simulink model "Mission_Server_Swarm_2QDrone_FrSky"  (Simulink 10.1)
settings: Solver=ode2  StartTime=0.0  StopTime=inf  FixedStep=0.001  RelTol=1e-3  EnableMultiTasking=on
undefined symbols (not defined in the file): datetime, Host, m, qc_get_step_size, saved_data
libraries: quarc_library x33, simulink x7
(part 2 of 2)

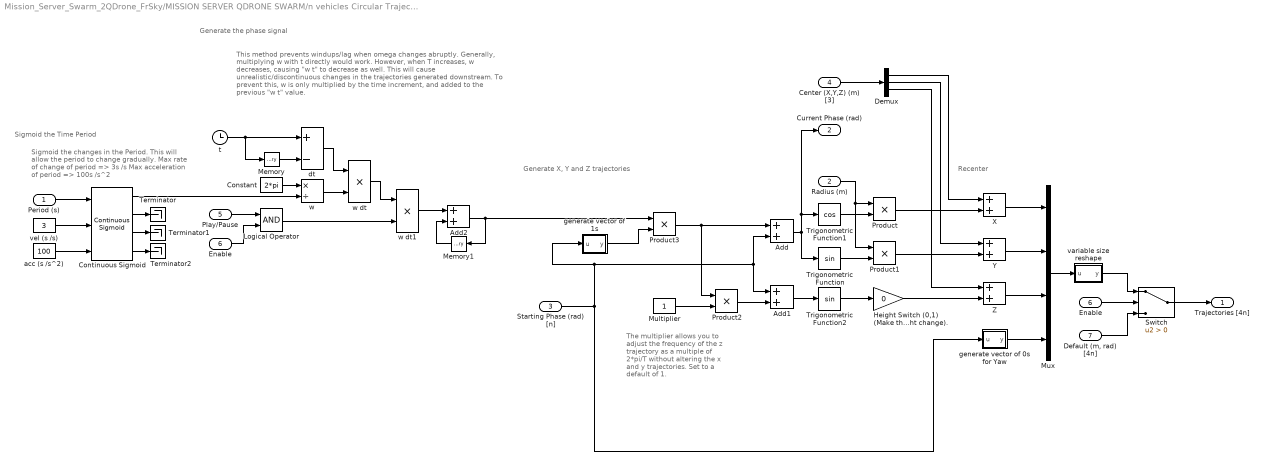
== system Mission_Server_Swarm_2QDrone_FrSky/MISSION SERVER QDRONE SWARM/n vehicles Circular Trajectories ==
  note: Recenter
  note: Generate X, Y and Z trajectories
  note: Generate the phase signal
  note: Sigmoid the changes in the Period. This will
      | allow the period to change gradually.
      | Max rate of change of period => 3s /s
      | Max acceleration of period => 100s /s^2
  note: Sigmoid the Time Period
  note: The multiplier allows you to adjust the frequency of the z trajectory as a multiple of 2*pi/T without altering the x and y trajectories. Set to a default of 1.
  note: This method prevents windups/lag when omega changes abruptly. Generally, multiplying w with t directly would work. However, when T increases, w decreases, causing "w t" to decrease as well. This will cause unrealistic/discontinuous changes in the trajectories generated downstream.
      |
      | To prevent this, w is only multiplied by the time increment, and added to the previous "w t" value.
  Period (s) : Inport
  Radius (m) : Inport  Port=2
  Starting Phase (rad) [n] : Inport  Port=3
  Center (X,Y,Z) (m) [3] : Inport  Port=4
  Play/Pause : Inport  Port=5
  Enable : Inport  Port=6
  "Default (m, rad) [4n]" : Inport  Port=7
  " Enable " : InportShadow  Port=6
  Add : Sum
  Add1 : Sum
  Add2 : Sum
  Constant : Constant  Value=2*pi
  Continuous Sigmoid : quarc_library/Sources/Sigmoids/Continuous Sigmoid  params_source=External (input ports)  max_velocity=2  max_acceleration=10  initial_position=10  initial_velocity=0  hold_off=0.5  input_sample_time=-1  output_sample_time=qc_get_step_size
      settings: SourceProductName=QUARC Targets
  Demux : Demux  Outputs=3
  Height Switch (0,1) (Make this 0 to disable height change). : Gain  Gain=0
  Logical Operator : Logic  AllPortsSameDT=off  OutDataTypeStr=boolean
  Memory : Memory
  Memory1 : Memory
  Multiplier : Constant
  Mux : Mux
  Product{,1..3} (4 alike) : Product
  Switch : Switch  Criteria=u2 > Threshold
  Terminator : Terminator
  Terminator1 : Terminator
  Terminator2 : Terminator
  Trigonometric Function : Trigonometry
  Trigonometric Function1 : Trigonometry  Operator=cos
  Trigonometric Function2 : Trigonometry
  X : Sum
  Y : Sum
  Z : Sum
  acc (s /s^2) : Constant  Value=100
  dt : Sum  Inputs=+-
  generate vector of 0s for Yaw : MATLAB Function  TreatAsAtomicUnit=on
  generate vector of 1s : MATLAB Function  TreatAsAtomicUnit=on
  t : Clock
  variable size reshape : MATLAB Function  TreatAsAtomicUnit=on
  vel (s /s) : Constant  Value=3
  w : Product  Inputs=*/
  w dt : Product
  w dt1 : Product
  Trajectories [4n] : Outport  VectorParamsAs1DForOutWhenUnconnected=off
  Current Phase (rad) : Outport  Port=2  VectorParamsAs1DForOutWhenUnconnected=off
  wires:
  Trigonometric Function/1 -> Product1/2
  Trigonometric Function1/1 -> Product/2
  Height Switch (0,1) (Make this 0 to disable height change)./1 -> Z/2
  Product1/1 -> Y/2
  Product/1 -> X/2
  Radius (m)/1 -> Product/1, Product1/1
  generate vector of 0s for Yaw/1(y) -> Mux/4
  Continuous Sigmoid/4 -> Terminator2/1
  Period (s)/1 -> Continuous Sigmoid/1
  Continuous Sigmoid/2 -> Terminator/1
  Continuous Sigmoid/3 -> Terminator1/1
  acc (s /s^2)/1 -> Continuous Sigmoid/3
  vel (s /s)/1 -> Continuous Sigmoid/2
  Add1/1 -> Trigonometric Function2/1
  Multiplier/1 -> Product2/2
  Starting Phase (rad) [n]/1 -> generate vector of 1s/1(u), Add/2, Add1/1, generate vector of 0s for Yaw/1(u)
  Add2/1 -> Product3/1, Memory1/1
  Add/1 -> Current Phase (rad)/1, Trigonometric Function1/1, Trigonometric Function/1
  Center (X,Y,Z) (m) [3]/1 -> Demux/1
  Demux/2 -> Y/1
  Demux/1 -> X/1
  Trigonometric Function2/1 -> Height Switch (0,1) (Make this 0 to disable height change)./1
  Demux/3 -> Z/1
  X/1 -> Mux/1
  Y/1 -> Mux/2
  Z/1 -> Mux/3
  Memory/1 -> dt/2
  w dt/1 -> w dt1/1
  w dt1/1 -> Add2/1
  Constant/1 -> w/1
  Memory1/1 -> Add2/2
  w/1 -> w dt/2
  Continuous Sigmoid/1 -> w/2
  t/1 -> Memory/1, dt/1
  dt/1 -> w dt/1
  Mux/1 -> variable size reshape/1(u)
  Switch/1 -> Trajectories [4n]/1
  "Default (m, rad) [4n]"/1 -> Switch/3
  Enable/1 -> Switch/2
  Play/Pause/1 -> Logical Operator/1
  " Enable "/1 -> Logical Operator/2
  Logical Operator/1 -> w dt1/2
  Product3/1 -> Add/1, Product2/1
  variable size reshape/1(y) -> Switch/1
  generate vector of 1s/1(y) -> Product3/2
  Product2/1 -> Add1/2

== system Mission_Server_Swarm_2QDrone_FrSky/MISSION SERVER QDRONE SWARM/Calculate Home Pose V1/Enabled Subsystem ==
  "Pose (m, rad ) [4] " : Inport
  Enable : EnablePort
  "Home Pose (m, rad ) [4]" : Outport  VectorParamsAs1DForOutWhenUnconnected=off
  wires:
  "Pose (m, rad ) [4] "/1 -> "Home Pose (m, rad ) [4]"/1

== system Mission_Server_Swarm_2QDrone_FrSky/MISSION SERVER QDRONE SWARM/Calculate Home Pose V2/Enabled Subsystem ==
  "Pose (m, rad ) [4] " : Inport
  Enable : EnablePort
  "Home Pose (m, rad ) [4]" : Outport  VectorParamsAs1DForOutWhenUnconnected=off
  wires:
  "Pose (m, rad ) [4] "/1 -> "Home Pose (m, rad ) [4]"/1

== system Mission_Server_Swarm_2QDrone_FrSky/MISSION SERVER QDRONE SWARM/Calculate Home Pose V7/Enabled Subsystem ==
  "Pose (m, rad ) [4] " : Inport
  Enable : EnablePort
  "Home Pose (m, rad ) [4]" : Outport  VectorParamsAs1DForOutWhenUnconnected=off
  wires:
  "Pose (m, rad ) [4] "/1 -> "Home Pose (m, rad ) [4]"/1

== system Mission_Server_Swarm_2QDrone_FrSky/MISSION SERVER QDRONE SWARM/Communications Check/Triggered Subsystem ==
  note: This looks for the first falling edge to trigger a communication issue,
      | because the mission server model starts first.
  Trigger : TriggerPort  TriggerType=falling  VariantControl=Variant
  Add : Sum
  Compare To Constant : simulink/Logic and Bit Operations/Compare To Constant  relop=>=  const=1  OutDataTypeStr=boolean
  Constant : Constant
  Memory : Memory  InheritSampleTime=on
  Communication Issue (0,1) : Outport  InitialOutput=0  VectorParamsAs1DForOutWhenUnconnected=off
  wires:
  Constant/1 -> Add/1
  Memory/1 -> Add/2
  Add/1 -> Compare To Constant/1, Memory/1
  Compare To Constant/1 -> Communication Issue (0,1)/1

== system Mission_Server_Swarm_2QDrone_FrSky/MISSION SERVER QDRONE SWARM/Communications Check/Triggered Subsystem1 ==
  note: This looks for the first falling edge to trigger a communication issue,
      | because the mission server model starts first.
  Trigger : TriggerPort  TriggerType=falling  VariantControl=Variant
  Add : Sum
  Compare To Constant : simulink/Logic and Bit Operations/Compare To Constant  relop=>=  const=1  OutDataTypeStr=boolean
  Constant : Constant
  Memory : Memory  InheritSampleTime=on
  Communication Issue (0,1) : Outport  InitialOutput=0  VectorParamsAs1DForOutWhenUnconnected=off
  wires:
  Compare To Constant/1 -> Communication Issue (0,1)/1
  Add/1 -> Memory/1, Compare To Constant/1
  Memory/1 -> Add/2
  Constant/1 -> Add/1

== system Mission_Server_Swarm_2QDrone_FrSky/MISSION SERVER QDRONE SWARM/Data Server (Localization) /Convention Correction (Motive Frame to Research Studio Frame) - Drone 1 ==
  note: MF_R_RSF
  note: This subsystem converts measurements in the Motive Frame (MF)(raw optitrack) into the Research Studio Frame (RSF).
  note: RSF_R_MF
  note: XYZ in MF
  note: RPY in MF
  note: position
  note: attitude
  note: XYZ in RSF
  note: RPY in RSF
  xyz_MF (m) [3] : Inport
  rot_MF (rad) [3] : Inport  Port=2
  Inverse of  Orthonormal  Matrix is its  Transpose : Math  Operator=transpose  SignedPower=on  SaturateOnIntegerOverflow=on
  Prevent Gimbal Lock : Subsystem
  Product : Product  Multiplication=Matrix(*)
  Product1 : Product  Multiplication=Matrix(*)
  Rotate Basis from  RSF to MF : Constant  Value=[0 -1 0;0 0 1;-1 0 0]
  xyz_RSF (m) [3] : Outport  VectorParamsAs1DForOutWhenUnconnected=off
  rot_RSF (rad) [3] : Outport  Port=2  VectorParamsAs1DForOutWhenUnconnected=off
  wires:
  Rotate Basis from  RSF to MF/1 -> Inverse of  Orthonormal  Matrix is its  Transpose/1
  xyz_MF (m) [3]/1 -> Product1/2
  Inverse of  Orthonormal  Matrix is its  Transpose/1 -> Product1/1, Product/1
  rot_MF (rad) [3]/1 -> Product/2
  Product1/1 -> xyz_RSF (m) [3]/1
  Product/1 -> Prevent Gimbal Lock/1(Attitude (rad) [3])
  Prevent Gimbal Lock/1("Attitude (rad) [3] ") -> rot_RSF (rad) [3]/1

== system Mission_Server_Swarm_2QDrone_FrSky/MISSION SERVER QDRONE SWARM/Data Server (Localization) /Convention Correction (Motive Frame to Research Studio Frame) - Drone 2 ==
  note: RPY in RSF
  note: XYZ in RSF
  note: attitude
  note: position
  note: RPY in MF
  note: XYZ in MF
  note: RSF_R_MF
  note: This subsystem converts measurements in the Motive Frame (MF)(raw optitrack) into the Research Studio Frame (RSF).
  note: MF_R_RSF
  xyz_MF (m) [3] : Inport
  rot_MF (rad) [3] : Inport  Port=2
  Inverse of  Orthonormal  Matrix is its  Transpose : Math  Operator=transpose  SignedPower=on  SaturateOnIntegerOverflow=on
  Prevent Gimbal Lock : Subsystem
  Product : Product  Multiplication=Matrix(*)
  Product1 : Product  Multiplication=Matrix(*)
  Rotate Basis from  RSF to MF : Constant  Value=[0 -1 0;0 0 1;-1 0 0]
  xyz_RSF (m) [3] : Outport  VectorParamsAs1DForOutWhenUnconnected=off
  rot_RSF (rad) [3] : Outport  Port=2  VectorParamsAs1DForOutWhenUnconnected=off
  wires:
  Prevent Gimbal Lock/1("Attitude (rad) [3] ") -> rot_RSF (rad) [3]/1
  Product/1 -> Prevent Gimbal Lock/1(Attitude (rad) [3])
  Product1/1 -> xyz_RSF (m) [3]/1
  rot_MF (rad) [3]/1 -> Product/2
  Inverse of  Orthonormal  Matrix is its  Transpose/1 -> Product/1, Product1/1
  xyz_MF (m) [3]/1 -> Product1/2
  Rotate Basis from  RSF to MF/1 -> Inverse of  Orthonormal  Matrix is its  Transpose/1

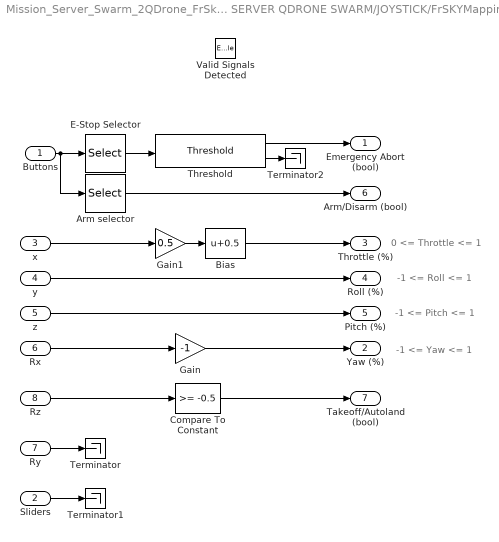
== system Mission_Server_Swarm_2QDrone_FrSky/MISSION SERVER QDRONE SWARM/JOYSTICK/FrSKYMapping ==
  note: -1 <= Pitch <= 1
  note: -1 <= Roll <= 1
  note: 0 <= Throttle <= 1
  note: -1 <= Yaw <= 1
  Buttons : Inport
  Sliders : Inport  Port=2
  x : Inport  Port=3
  y : Inport  Port=4
  z : Inport  Port=5
  Rx : Inport  Port=6
  Ry : Inport  Port=7
  Rz : Inport  Port=8
  Valid Signals Detected : EnablePort
  Arm selector : Selector  InputPortWidth=32  IndexOptions=Index vector (dialog)  Indices=[2]  OutputSizes=1
  Bias : Bias  Bias=0.5
  Compare To Constant : simulink/Logic and Bit Operations/Compare To Constant  relop=>=  const=-0.5  OutDataTypeStr=boolean
  E-Stop Selector : Selector  InputPortWidth=32  IndexOptions=Index vector (dialog)  Indices=[1]  OutputSizes=1
  Gain : Gain  Gain=-1
  Gain1 : Gain  Gain=0.5
  Terminator : Terminator
  Terminator1 : Terminator
  Terminator2 : Terminator
  Threshold : quarc_library/Discontinuities/Threshold  operator=>=  param_src=Specify via dialog  threshold=0.5  duration=0.2
      settings: SourceProductName=QUARC Targets
  Emergency Abort (bool) : Outport  VectorParamsAs1DForOutWhenUnconnected=off
  Yaw (%) : Outport  Port=2  VectorParamsAs1DForOutWhenUnconnected=off
  Throttle (%) : Outport  Port=3  VectorParamsAs1DForOutWhenUnconnected=off
  Roll (%) : Outport  Port=4  VectorParamsAs1DForOutWhenUnconnected=off
  Pitch (%) : Outport  Port=5  VectorParamsAs1DForOutWhenUnconnected=off
  "Arm/Disarm (bool) " : Outport  Port=6  VectorParamsAs1DForOutWhenUnconnected=off
  Takeoff/Autoland (bool) : Outport  Port=7  VectorParamsAs1DForOutWhenUnconnected=off
  wires:
  Bias/1 -> Throttle (%)/1
  Gain1/1 -> Bias/1
  Gain/1 -> Yaw (%)/1
  Threshold/2 -> Terminator2/1
  Threshold/1 -> Emergency Abort (bool)/1
  Compare To Constant/1 -> Takeoff/Autoland (bool)/1
  Rz/1 -> Compare To Constant/1
  E-Stop Selector/1 -> Threshold/1
  Sliders/1 -> Terminator1/1
  Ry/1 -> Terminator/1
  Rx/1 -> Gain/1
  z/1 -> Pitch (%)/1
  y/1 -> Roll (%)/1
  x/1 -> Gain1/1
  Arm selector/1 -> "Arm/Disarm (bool) "/1
  Buttons/1 -> E-Stop Selector/1, Arm selector/1

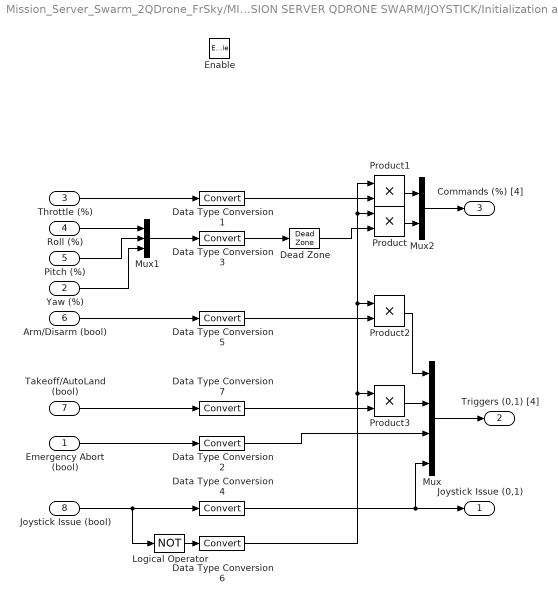
== system Mission_Server_Swarm_2QDrone_FrSky/MISSION SERVER QDRONE SWARM/JOYSTICK/Initialization and Conditioning ==
  Emergency Abort (bool) : Inport
  Yaw (%) : Inport  Port=2
  Throttle (%) : Inport  Port=3
  Roll (%) : Inport  Port=4
  Pitch (%) : Inport  Port=5
  Arm/Disarm (bool) : Inport  Port=6
  Takeoff/AutoLand (bool) : Inport  Port=7
  Joystick Issue (bool) : Inport  Port=8
  Enable : EnablePort  StatesWhenEnabling=reset
  Data Type Conversion{1..7} (7 alike) : DataTypeConversion
  Dead Zone : DeadZone  LowerValue=-0.01  UpperValue=0.01  SaturateOnIntegerOverflow=on
  Logical Operator : Logic  Operator=NOT  AllPortsSameDT=off  OutDataTypeStr=boolean
  Mux : Mux
  Mux1 : Mux  Inputs=3
  Mux2 : Mux  Inputs=2
  Product{,1..3} (4 alike) : Product
  Joystick Issue (0,1) : Outport  InitialOutput=0  VectorParamsAs1DForOutWhenUnconnected=off
  Triggers (0,1) [4] : Outport  Port=2  InitialOutput=0  VectorParamsAs1DForOutWhenUnconnected=off
  Commands (%) [4] : Outport  Port=3  InitialOutput=0  VectorParamsAs1DForOutWhenUnconnected=off
  wires:
  Mux2/1 -> Commands (%) [4]/1
  Data Type Conversion7/1 -> Product3/2
  Product3/1 -> Mux/2
  Takeoff/AutoLand (bool)/1 -> Data Type Conversion7/1
  Data Type Conversion5/1 -> Product2/2
  Product2/1 -> Mux/1
  Data Type Conversion6/1 -> Product3/1, Product2/1, Product/1, Product1/1
  Dead Zone/1 -> Product/2
  Data Type Conversion1/1 -> Product1/2
  Product1/1 -> Mux2/1
  Product/1 -> Mux2/2
  Logical Operator/1 -> Data Type Conversion6/1
  Data Type Conversion2/1 -> Mux/3
  Mux/1 -> Triggers (0,1) [4]/1
  Arm/Disarm (bool)/1 -> Data Type Conversion5/1
  Data Type Conversion3/1 -> Dead Zone/1
  Emergency Abort (bool)/1 -> Data Type Conversion2/1
  Data Type Conversion4/1 -> Joystick Issue (0,1)/1, Mux/4
  Yaw (%)/1 -> Mux1/3
  Pitch (%)/1 -> Mux1/2
  Roll (%)/1 -> Mux1/1
  Throttle (%)/1 -> Data Type Conversion1/1
  Mux1/1 -> Data Type Conversion3/1
  Joystick Issue (bool)/1 -> Logical Operator/1, Data Type Conversion4/1

== system Mission_Server_Swarm_2QDrone_FrSky/MISSION SERVER QDRONE SWARM/JOYSTICK/Pulse Check ==
  note: For this subsystem we will count the number of new pulses. The data can be considered enabled once the count of new signals has gone beyond 1. This will enable the Initializing and conditioning subsystem.
  new : Inport
  Compare : quarc_library/Logic Operations/Compare  operator=>=  output_data_type=boolean
      settings: SourceProductName=QUARC Targets
  Pulse Check : Constant
  "pulse count " : Subsystem  TreatAsAtomicUnit=on
  signal enable : Outport  InitialOutput=0  VectorParamsAs1DForOutWhenUnconnected=off
  wires:
  Compare/1 -> signal enable/1
  Pulse Check/1 -> Compare/2
  new/1 -> "pulse count "/Trigger
  "pulse count "/1(Number of Pulses) -> Compare/1

== system Mission_Server_Swarm_2QDrone_FrSky/MISSION SERVER QDRONE SWARM/Data Server (Localization) /Convention Correction (Motive Frame to Research Studio Frame) - Drone 1/Prevent Gimbal Lock ==
  note: Remapping the rotation order to prevent gimbal lock
      | in heading/yaw due to Euler singularity condition
  Attitude (rad) [3] : Inport
  Demux : Demux  Outputs=3
  Euler Angles from Rotation Matrix (Relative ZYX) : quarc_library/Math Operations/Matrices/Euler Angles from Rotation Matrix  menu_order=Relative Z-Y-X
      settings: SourceProductName=QUARC Targets
  Euler Angles to Rotation Matrix (Relative YZX) : quarc_library/Math Operations/Matrices/Euler Angles to Rotation Matrix  menu_order=Relative Y-Z-X
      settings: SourceProductName=QUARC Targets
  Mux : Mux  Inputs=3
  "Attitude (rad) [3] " : Outport  VectorParamsAs1DForOutWhenUnconnected=off
  wires:
  Euler Angles from Rotation Matrix (Relative ZYX)/2 -> Mux/2
  Euler Angles from Rotation Matrix (Relative ZYX)/1 -> Mux/3
  Euler Angles from Rotation Matrix (Relative ZYX)/3 -> Mux/1
  Euler Angles to Rotation Matrix (Relative YZX)/1 -> Euler Angles from Rotation Matrix (Relative ZYX)/1
  Attitude (rad) [3]/1 -> Demux/1
  Mux/1 -> "Attitude (rad) [3] "/1
  Demux/2 -> Euler Angles to Rotation Matrix (Relative YZX)/1
  Demux/3 -> Euler Angles to Rotation Matrix (Relative YZX)/2
  Demux/1 -> Euler Angles to Rotation Matrix (Relative YZX)/3

== system Mission_Server_Swarm_2QDrone_FrSky/MISSION SERVER QDRONE SWARM/Data Server (Localization) /Convention Correction (Motive Frame to Research Studio Frame) - Drone 2/Prevent Gimbal Lock ==
  note: Remapping the rotation order to prevent gimbal lock
      | in heading/yaw due to Euler singularity condition
  Attitude (rad) [3] : Inport
  Demux : Demux  Outputs=3
  Euler Angles from Rotation Matrix (Relative ZYX) : quarc_library/Math Operations/Matrices/Euler Angles from Rotation Matrix  menu_order=Relative Z-Y-X
      settings: SourceProductName=QUARC Targets
  Euler Angles to Rotation Matrix (Relative YZX) : quarc_library/Math Operations/Matrices/Euler Angles to Rotation Matrix  menu_order=Relative Y-Z-X
      settings: SourceProductName=QUARC Targets
  Mux : Mux  Inputs=3
  "Attitude (rad) [3] " : Outport  VectorParamsAs1DForOutWhenUnconnected=off
  wires:
  Demux/1 -> Euler Angles to Rotation Matrix (Relative YZX)/3
  Demux/3 -> Euler Angles to Rotation Matrix (Relative YZX)/2
  Demux/2 -> Euler Angles to Rotation Matrix (Relative YZX)/1
  Mux/1 -> "Attitude (rad) [3] "/1
  Attitude (rad) [3]/1 -> Demux/1
  Euler Angles to Rotation Matrix (Relative YZX)/1 -> Euler Angles from Rotation Matrix (Relative ZYX)/1
  Euler Angles from Rotation Matrix (Relative ZYX)/3 -> Mux/1
  Euler Angles from Rotation Matrix (Relative ZYX)/1 -> Mux/3
  Euler Angles from Rotation Matrix (Relative ZYX)/2 -> Mux/2

== system Mission_Server_Swarm_2QDrone_FrSky/MISSION SERVER QDRONE SWARM/JOYSTICK/Pulse Check/pulse count  ==
  Trigger : TriggerPort  TriggerType=either  VariantControl=Variant
  Constant1 : Constant  Value=0
  Increment Stored Integer : simulink/Additional Math & Discrete/Additional Math: Increment - Decrement/Increment Stored Integer
  Sum : Sum  Inputs=|++
  Unit Delay : UnitDelay  SampleTime=-1  HasFrameUpgradeWarning=on
  Number of Pulses : Outport  VectorParamsAs1DForOutWhenUnconnected=off
  wires:
  Constant1/1 -> Sum/1
  Sum/1 -> Increment Stored Integer/1
  Unit Delay/1 -> Sum/2
  Increment Stored Integer/1 -> Unit Delay/1, Number of Pulses/1

== matlab function MISSION SERVER QDRONE SWARM/n vehicles Circular Trajectories/generate vector of 0s for Yaw ==
  data: u input double; y output double
function y = fcn(u)

y = 0.*u;

== matlab function MISSION SERVER QDRONE SWARM/n vehicles Circular Trajectories/generate vector of 1s ==
  data: u input double; y output double
function y = fcn(u)

y = 0.*u + 1;

== matlab function MISSION SERVER QDRONE SWARM/n vehicles Circular Trajectories/variable size reshape ==
  data: u input double; y output double
function y = fcn(u)
y = u;
num = length(u)/4;
for i = 1:4
    for j = 1:num
        y(4*(j-1) + i) = u(j + num*(i-1));
    end
end

== matlab function Communication V1/Detect Communication loss/MATLAB Function ==
  data: time input double; stream_connection_loss output double; state input double; error input double
function stream_connection_loss  = fcn(time, state, error)

stream_connection_loss = 0;
if time > 1
    if ~((state == 2)&&(error >= 0))
        % stream connection is not established correctly
        stream_connection_loss = 1;
    end
end

== matlab function Communication V2/Detect Communication loss/MATLAB Function ==
  data: time input double; stream_connection_loss output double; state input double; error input double
function stream_connection_loss  = fcn(time, state, error)

stream_connection_loss = 0;
if time > 1
    if ~((state == 2)&&(error >= 0))
        % stream connection is not established correctly
        stream_connection_loss = 1;
    end
end

== matlab function MISSION SERVER QDRONE SWARM/Extract Vehicle Data 7/Extract Object Data ==
  data: data input double; position output double; orientation output double; index input double; tracking output double
function [position, orientation, tracking] = fcn(data, index)

n = length(data)/7;

if (index<=0)||(index>n)
    position = zeros(1,3); orientation = zeros(1,3); tracking = 0;
else
    position = [data(index*3-2), data(index*3-1), data(index*3)];
    orientation = [data((index+n)*3 - 2), data((index+n)*3 - 1), data((index+n)*3)];
    tracking = data(index + (n*6));
end

== matlab function MISSION SERVER QDRONE SWARM/Extract Vehicle Data 1/Extract Object Data ==
  data: data input double; position output double; orientation output double; index input double; tracking output double
function [position, orientation, tracking] = fcn(data, index)

n = length(data)/7;

if (index<=0)||(index>n)
    position = zeros(1,3); orientation = zeros(1,3); tracking = 0;
else
    position = [data(index*3-2), data(index*3-1), data(index*3)];
    orientation = [data((index+n)*3 - 2), data((index+n)*3 - 1), data((index+n)*3)];
    tracking = data(index + (n*6));
end

== matlab function MISSION SERVER QDRONE SWARM/Extract Vehicle Data 2/Extract Object Data ==
  data: data input double; position output double; orientation output double; index input double; tracking output double
function [position, orientation, tracking] = fcn(data, index)

n = length(data)/7;

if (index<=0)||(index>n)
    position = zeros(1,3); orientation = zeros(1,3); tracking = 0;
else
    position = [data(index*3-2), data(index*3-1), data(index*3)];
    orientation = [data((index+n)*3 - 2), data((index+n)*3 - 1), data((index+n)*3)];
    tracking = data(index + (n*6));
end
